simulink model "Ejer2_EnfriamientoNewton"  (R2023b)
settings: Solver=FixedStepDiscrete  StartTime=0  StopTime=15  FixedStep=1  RelTol=1e-3
undefined symbols (not defined in the file): k, S, t0
settings Model: Creator=alfre  LastModifiedBy=alfre

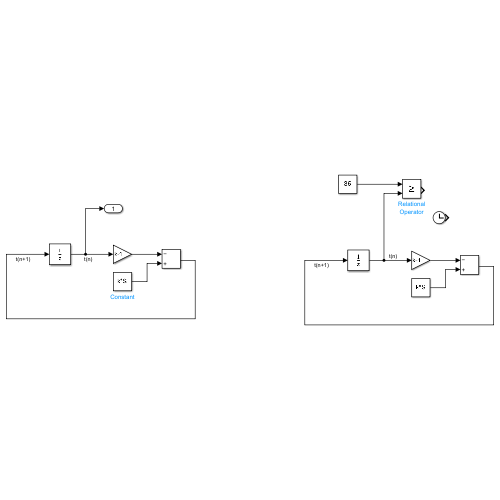
[thumbnail: Simulink's stored preview of the top-level diagram]
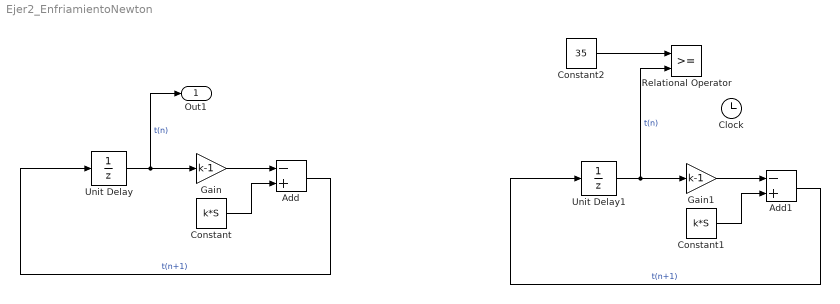
== system Ejer2_EnfriamientoNewton ==
  Add : Sum  Inputs=-+
  Add1 : Sum  Inputs=-+
  Clock : Clock
  Constant : Constant  Value=k*S
  Constant1 : Constant  Value=k*S
  Constant2 : Constant  Value=35
  Gain : Gain  Gain=k-1
  Gain1 : Gain  Gain=k-1
  Relational Operator : RelationalOperator  OutDataTypeStr=boolean  RndMeth=Simplest  InputSameDT=off
  Unit Delay : UnitDelay  InitialCondition=t0  SampleTime=-1  HasFrameUpgradeWarning=on
  Unit Delay1 : UnitDelay  InitialCondition=t0  SampleTime=-1  HasFrameUpgradeWarning=on
  Out1 : Outport
  wires:
  Unit Delay/1 -> Out1/1, Gain/1  "t(n)"
  Add/1 -> Unit Delay/1  "t(n+1)"
  Constant/1 -> Add/2
  Gain/1 -> Add/1
  Unit Delay1/1 -> Relational Operator/2, Gain1/1  "t(n)"
  Constant1/1 -> Add1/2
  Add1/1 -> Unit Delay1/1  "t(n+1)"
  Gain1/1 -> Add1/1
  Constant2/1 -> Relational Operator/1
